simulink model "dcm"  (R2015a)
settings: Solver=ode45  StartTime=0.0  StopTime=10.0  RelTol=1e-3
libraries: nesl_utility x16, fl_lib x15, elec_lib x1
settings Model: Creator=tomas  LastModifiedBy=tomas

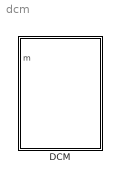
== system dcm ==
  DCM : Subsystem

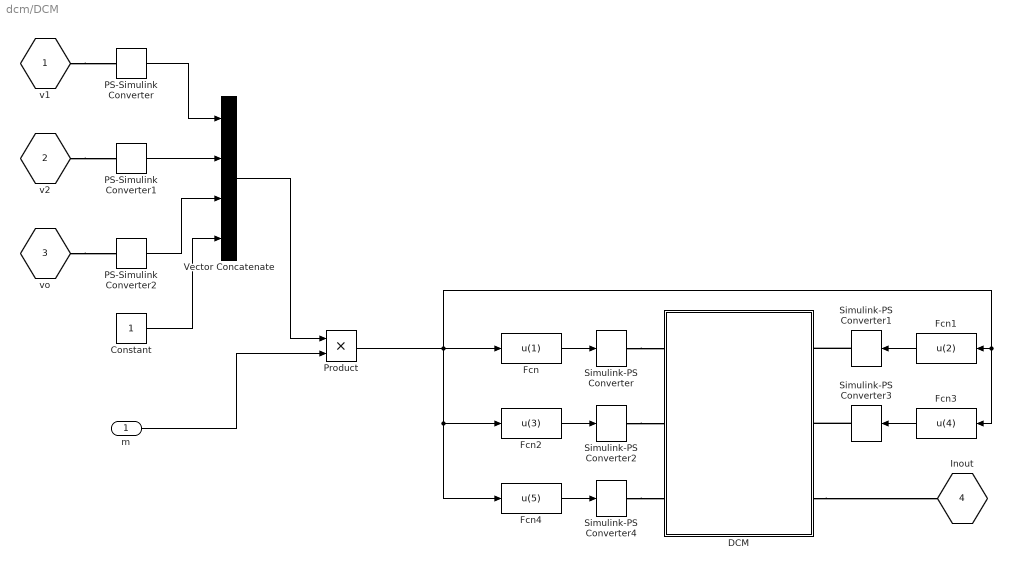
== system dcm/DCM ==
  m : Inport
  Constant : Constant
  DCM : Subsystem
  Fcn : Fcn  Expr=u(1)
  Fcn1 : Fcn  Expr=u(2)
  Fcn2 : Fcn  Expr=u(3)
  Fcn3 : Fcn  Expr=u(4)
  Fcn4 : Fcn  Expr=u(5)
  PS-Simulink Converter : nesl_utility/PS-Simulink Converter  PhysicalDomain=network_engine_domain  SubClassName=ps_output  LeftPortType=input  RightPortType=output  PseudoPeriodic=off  Frequencies=[]  Unit=1  AffineConversion=off
  PS-Simulink Converter1 : nesl_utility/PS-Simulink Converter  PhysicalDomain=network_engine_domain  SubClassName=ps_output  LeftPortType=input  RightPortType=output  PseudoPeriodic=off  Frequencies=[]  Unit=1  AffineConversion=off
  PS-Simulink Converter2 : nesl_utility/PS-Simulink Converter  PhysicalDomain=network_engine_domain  SubClassName=ps_output  LeftPortType=input  RightPortType=output  PseudoPeriodic=off  Frequencies=[]  Unit=1  AffineConversion=off
  Product : Product
  Simulink-PS Converter{,1..4} (5 alike) : nesl_utility/Simulink-PS Converter  PhysicalDomain=network_engine_domain  SubClassName=ps_input  LeftPortType=input  RightPortType=output  PseudoPeriodic=off  Frequencies=[]  NoiseDistribution=none  NoiseParameters=[]  Unit=1  AffineConversion=off  InputFiltering=off  SimscapeFilterOrder=1  InputFilterTimeConstant=0.001  UdotUserProvided=1
  Vector Concatenate : Concatenate  NumInputs=4
  "v1 " : PMIOPort  Port=1  Side=Left
  v2 : PMIOPort  Port=2  Side=Right
  vo : PMIOPort  Port=3  Side=Left
  Inout : PMIOPort  Port=4  Side=Right
  wires:
  m/1 -> Product/2
  Fcn4/1 -> Simulink-PS Converter4/1
  Constant/1 -> Vector Concatenate/4
  Product/1 -> Fcn3/1, Fcn1/1, Fcn2/1, Fcn4/1, Fcn/1
  Fcn2/1 -> Simulink-PS Converter2/1
  PS-Simulink Converter/1 -> Vector Concatenate/1
  PS-Simulink Converter2/1 -> Vector Concatenate/3
  Fcn1/1 -> Simulink-PS Converter1/1
  PS-Simulink Converter1/1 -> Vector Concatenate/2
  Fcn/1 -> Simulink-PS Converter/1
  Vector Concatenate/1 -> Product/1
  Fcn3/1 -> Simulink-PS Converter3/1
  connections:
  Simulink-PS Converter2/RConn1 -- DCM/LConn2
  DCM/RConn3 -- Inout/RConn1
  Simulink-PS Converter3/RConn1 -- DCM/RConn2
  vo/RConn1 -- PS-Simulink Converter2/LConn1
  Simulink-PS Converter4/RConn1 -- DCM/LConn3
  Simulink-PS Converter/RConn1 -- DCM/LConn1
  "v1 "/RConn1 -- PS-Simulink Converter/LConn1
  v2/RConn1 -- PS-Simulink Converter1/LConn1
  Simulink-PS Converter1/RConn1 -- DCM/RConn1

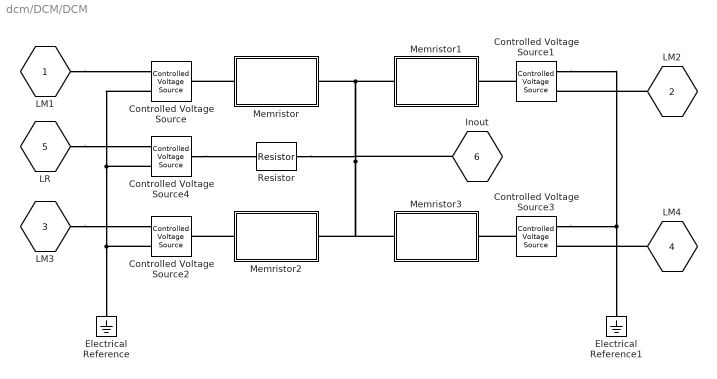
== system dcm/DCM/DCM ==
  Controlled Voltage Source{,1..4} (5 alike) : fl_lib/Electrical/Electrical Sources/Controlled Voltage Source
  Electrical Reference : fl_lib/Electrical/Electrical Elements/Electrical Reference
  Electrical Reference1 : fl_lib/Electrical/Electrical Elements/Electrical Reference
  Memristor : Subsystem  Tag=Memristor
  Memristor1 : Subsystem  Tag=Memristor
  Memristor2 : Subsystem  Tag=Memristor
  Memristor3 : Subsystem  Tag=Memristor
  Resistor : elec_lib/Passive Devices/Resistor  R=1 Ohm  noise_mode=0  Tdevice=25 C  sample_time=0.001 s  repeatability=1  auto_seed=970326661  user_seed=0
  LM1 : PMIOPort  Port=1  Side=Left
  LM2 : PMIOPort  Port=2  Side=Right
  LM3 : PMIOPort  Port=3  Side=Left
  LM4 : PMIOPort  Port=4  Side=Right
  LR : PMIOPort  Port=5  Side=Left
  Inout : PMIOPort  Port=6  Side=Right
  connections:
  LM2/RConn1 -- Controlled Voltage Source1/RConn1
  Controlled Voltage Source/RConn2 -- Controlled Voltage Source4/RConn2 -- Controlled Voltage Source2/RConn2 -- Electrical Reference/LConn1
  Controlled Voltage Source4/LConn1 -- Resistor/LConn1
  Memristor1/RConn1 -- Inout/RConn1 -- Resistor/RConn1 -- Memristor2/RConn1 -- Memristor3/RConn1 -- Memristor/RConn1
  Memristor2/LConn1 -- Controlled Voltage Source2/LConn1
  Controlled Voltage Source3/LConn1 -- Memristor3/LConn1
  Controlled Voltage Source1/RConn2 -- Controlled Voltage Source3/RConn2 -- Electrical Reference1/LConn1
  LM1/RConn1 -- Controlled Voltage Source/RConn1
  LM4/RConn1 -- Controlled Voltage Source3/RConn1
  LR/RConn1 -- Controlled Voltage Source4/RConn1
  LM3/RConn1 -- Controlled Voltage Source2/RConn1
  Memristor/LConn1 -- Controlled Voltage Source/LConn1
  Controlled Voltage Source1/LConn1 -- Memristor1/LConn1

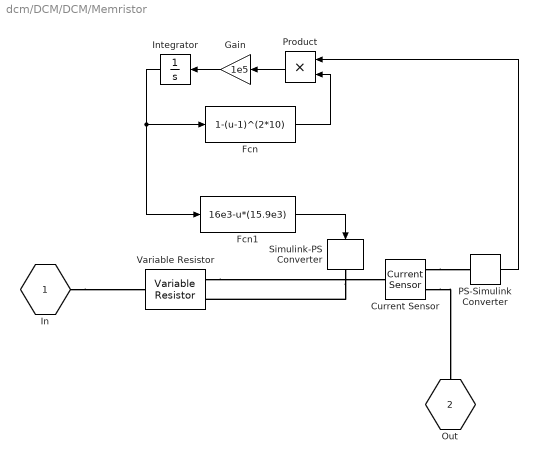
== system dcm/DCM/DCM/Memristor ==
  Current Sensor : fl_lib/Electrical/Electrical Sensors/Current Sensor
  Fcn : Fcn  Expr=1-(u-1)^(2*10)
  Fcn1 : Fcn  Expr=16e3-u*(15.9e3)
  Gain : Gain  Gain=1e5
  Integrator : Integrator  InitialCondition=0.3145
  PS-Simulink Converter : nesl_utility/PS-Simulink Converter  PhysicalDomain=network_engine_domain  SubClassName=ps_output  LeftPortType=input  RightPortType=output  PseudoPeriodic=off  Frequencies=[]  Unit=1  AffineConversion=off
  Product : Product
  Simulink-PS Converter : nesl_utility/Simulink-PS Converter  PhysicalDomain=network_engine_domain  SubClassName=ps_input  LeftPortType=input  RightPortType=output  PseudoPeriodic=off  Frequencies=[]  NoiseDistribution=none  NoiseParameters=[]  Unit=1  AffineConversion=off  InputFiltering=off  SimscapeFilterOrder=1  InputFilterTimeConstant=0.001  UdotUserProvided=1
  Variable Resistor : fl_lib/Electrical/Electrical Elements/Variable Resistor  Rmin=0 Ohm  i_specify=off  i_priority=High  i=0 A  v_specify=off  v_priority=High  v=0 V
  In : PMIOPort  Port=1  Side=Left
  Out : PMIOPort  Port=2  Side=Right
  wires:
  Gain/1 -> Integrator/1
  Product/1 -> Gain/1
  Integrator/1 -> Fcn1/1, Fcn/1
  Fcn/1 -> Product/2
  Fcn1/1 -> Simulink-PS Converter/1
  PS-Simulink Converter/1 -> Product/1
  connections:
  In/RConn1 -- Variable Resistor/RConn1
  Variable Resistor/LConn2 -- Current Sensor/LConn1
  Current Sensor/RConn1 -- PS-Simulink Converter/LConn1
  Simulink-PS Converter/RConn1 -- Variable Resistor/LConn1
  Current Sensor/RConn2 -- Out/RConn1

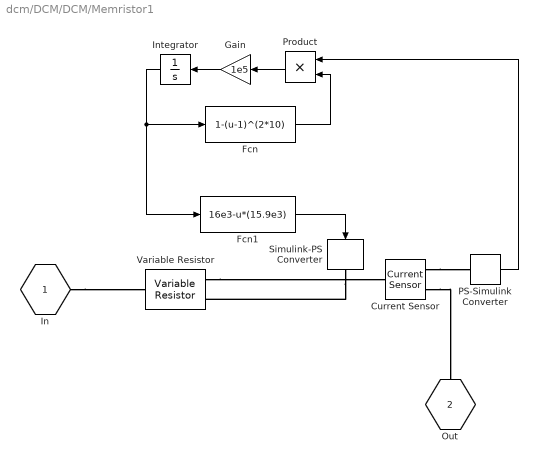
== system dcm/DCM/DCM/Memristor1 ==
  Current Sensor : fl_lib/Electrical/Electrical Sensors/Current Sensor
  Fcn : Fcn  Expr=1-(u-1)^(2*10)
  Fcn1 : Fcn  Expr=16e3-u*(15.9e3)
  Gain : Gain  Gain=1e5
  Integrator : Integrator  InitialCondition=0.3145
  PS-Simulink Converter : nesl_utility/PS-Simulink Converter  PhysicalDomain=network_engine_domain  SubClassName=ps_output  LeftPortType=input  RightPortType=output  PseudoPeriodic=off  Frequencies=[]  Unit=1  AffineConversion=off
  Product : Product
  Simulink-PS Converter : nesl_utility/Simulink-PS Converter  PhysicalDomain=network_engine_domain  SubClassName=ps_input  LeftPortType=input  RightPortType=output  PseudoPeriodic=off  Frequencies=[]  NoiseDistribution=none  NoiseParameters=[]  Unit=1  AffineConversion=off  InputFiltering=off  SimscapeFilterOrder=1  InputFilterTimeConstant=0.001  UdotUserProvided=1
  Variable Resistor : fl_lib/Electrical/Electrical Elements/Variable Resistor  Rmin=0 Ohm  i_specify=off  i_priority=High  i=0 A  v_specify=off  v_priority=High  v=0 V
  In : PMIOPort  Port=1  Side=Left
  Out : PMIOPort  Port=2  Side=Right
  wires:
  Gain/1 -> Integrator/1
  Product/1 -> Gain/1
  Integrator/1 -> Fcn1/1, Fcn/1
  Fcn/1 -> Product/2
  Fcn1/1 -> Simulink-PS Converter/1
  PS-Simulink Converter/1 -> Product/1
  connections:
  In/RConn1 -- Variable Resistor/RConn1
  Variable Resistor/LConn2 -- Current Sensor/LConn1
  Current Sensor/RConn1 -- PS-Simulink Converter/LConn1
  Simulink-PS Converter/RConn1 -- Variable Resistor/LConn1
  Current Sensor/RConn2 -- Out/RConn1

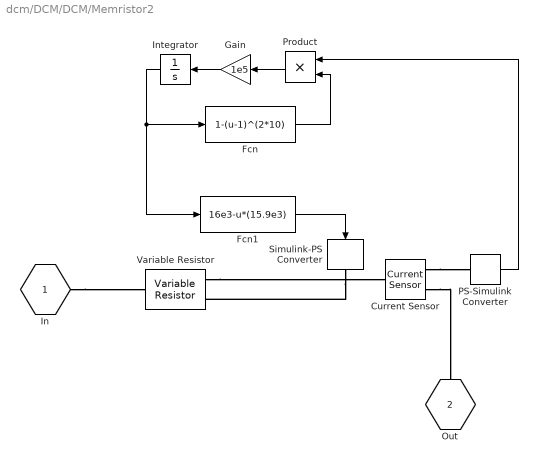
== system dcm/DCM/DCM/Memristor2 ==
  Current Sensor : fl_lib/Electrical/Electrical Sensors/Current Sensor
  Fcn : Fcn  Expr=1-(u-1)^(2*10)
  Fcn1 : Fcn  Expr=16e3-u*(15.9e3)
  Gain : Gain  Gain=1e5
  Integrator : Integrator  InitialCondition=0.3145
  PS-Simulink Converter : nesl_utility/PS-Simulink Converter  PhysicalDomain=network_engine_domain  SubClassName=ps_output  LeftPortType=input  RightPortType=output  PseudoPeriodic=off  Frequencies=[]  Unit=1  AffineConversion=off
  Product : Product
  Simulink-PS Converter : nesl_utility/Simulink-PS Converter  PhysicalDomain=network_engine_domain  SubClassName=ps_input  LeftPortType=input  RightPortType=output  PseudoPeriodic=off  Frequencies=[]  NoiseDistribution=none  NoiseParameters=[]  Unit=1  AffineConversion=off  InputFiltering=off  SimscapeFilterOrder=1  InputFilterTimeConstant=0.001  UdotUserProvided=1
  Variable Resistor : fl_lib/Electrical/Electrical Elements/Variable Resistor  Rmin=0 Ohm  i_specify=off  i_priority=High  i=0 A  v_specify=off  v_priority=High  v=0 V
  In : PMIOPort  Port=1  Side=Left
  Out : PMIOPort  Port=2  Side=Right
  wires:
  Gain/1 -> Integrator/1
  Product/1 -> Gain/1
  Integrator/1 -> Fcn1/1, Fcn/1
  Fcn/1 -> Product/2
  Fcn1/1 -> Simulink-PS Converter/1
  PS-Simulink Converter/1 -> Product/1
  connections:
  In/RConn1 -- Variable Resistor/RConn1
  Variable Resistor/LConn2 -- Current Sensor/LConn1
  Current Sensor/RConn1 -- PS-Simulink Converter/LConn1
  Simulink-PS Converter/RConn1 -- Variable Resistor/LConn1
  Current Sensor/RConn2 -- Out/RConn1

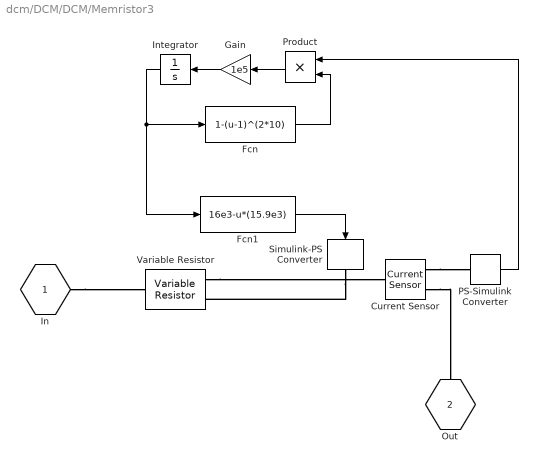
== system dcm/DCM/DCM/Memristor3 ==
  Current Sensor : fl_lib/Electrical/Electrical Sensors/Current Sensor
  Fcn : Fcn  Expr=1-(u-1)^(2*10)
  Fcn1 : Fcn  Expr=16e3-u*(15.9e3)
  Gain : Gain  Gain=1e5
  Integrator : Integrator  InitialCondition=0.3145
  PS-Simulink Converter : nesl_utility/PS-Simulink Converter  PhysicalDomain=network_engine_domain  SubClassName=ps_output  LeftPortType=input  RightPortType=output  PseudoPeriodic=off  Frequencies=[]  Unit=1  AffineConversion=off
  Product : Product
  Simulink-PS Converter : nesl_utility/Simulink-PS Converter  PhysicalDomain=network_engine_domain  SubClassName=ps_input  LeftPortType=input  RightPortType=output  PseudoPeriodic=off  Frequencies=[]  NoiseDistribution=none  NoiseParameters=[]  Unit=1  AffineConversion=off  InputFiltering=off  SimscapeFilterOrder=1  InputFilterTimeConstant=0.001  UdotUserProvided=1
  Variable Resistor : fl_lib/Electrical/Electrical Elements/Variable Resistor  Rmin=0 Ohm  i_specify=off  i_priority=High  i=0 A  v_specify=off  v_priority=High  v=0 V
  In : PMIOPort  Port=1  Side=Left
  Out : PMIOPort  Port=2  Side=Right
  wires:
  Gain/1 -> Integrator/1
  Product/1 -> Gain/1
  Integrator/1 -> Fcn1/1, Fcn/1
  Fcn/1 -> Product/2
  Fcn1/1 -> Simulink-PS Converter/1
  PS-Simulink Converter/1 -> Product/1
  connections:
  In/RConn1 -- Variable Resistor/RConn1
  Variable Resistor/LConn2 -- Current Sensor/LConn1
  Current Sensor/RConn1 -- PS-Simulink Converter/LConn1
  Simulink-PS Converter/RConn1 -- Variable Resistor/LConn1
  Current Sensor/RConn2 -- Out/RConn1
